simulink model "MPSK_basemodem"  (Simulink 9.2)
settings: Solver=VariableStepDiscrete  StartTime=0.0  StopTime=10  FixedStep=1/100000  RelTol=1e-3  AbsTol=1e-6
PreLoadFcn:
  | M=16;
libraries: commutil2 x2, commsink2 x2, commdigbbndpm3 x2, commchan3 x1, commrandsrc2 x1
settings Model: Creator=amoura  LastModifiedBy=nox
settings SolverCC: AutoScaleAbsTol=off
settings DataIOCC: LimitDataPoints=off
settings OptimizationCC: BlockReduction=off  BooleanDataType=off  ExpressionDepthLimit=2147483647  InitFltsAndDblsToZero=on
settings DebuggingCC: SaveWithParameterizedLinksMsg=none  SignalResolutionControl=TryResolveAllWithWarning  MultiTaskDSMMsg=warning  MultiTaskCondExecSysMsg=none
settings HardwareCC: TargetUnknown=on
settings RTWCC: TemplateMakefile=grt_unix.tmf
settings GRTTargetCC: TargetFcnLib=ansi_tfl_tmw.mat  ModelReferenceCompliant=off  MatFileLogging=off

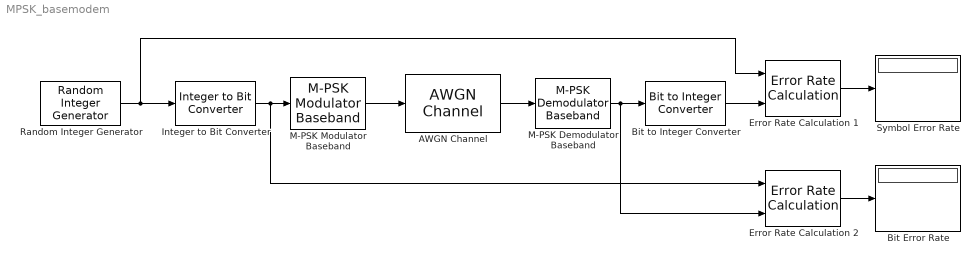
== system MPSK_basemodem ==
  AWGN Channel : commchan3/AWGN Channel  InputProcessing=Columns as channels (frame based)  seed=67  noiseMode="Signal to noise ratio  (Es/No)"  EbNodB=9.21  EsNodB=8  SNRdB=10  bitsPerSym=3  Ps=1  Tsym=1/1000  variance=1
  Bit Error Rate : Display
  Bit to Integer Converter : commutil2/Bit to Integer Converter  nbits=log2(M)  bitOrder=MSB first  signedOutputValues=Unsigned  outDtype=Inherit via internal rule  outDtypeSigned=Inherit via internal rule
  Error Rate Calculation 1 : commsink2/Error Rate Calculation  N=0  st_delay=0  cp_mode=Entire frame  subframe=[]  PMode=Port  WsName=ErrorVec  RsMode2=off  stop=off  numErr=100  maxBits=1e6
  Error Rate Calculation 2 : commsink2/Error Rate Calculation  N=0  st_delay=0  cp_mode=Entire frame  subframe=[]  PMode=Port  WsName=ErrorVec  RsMode2=off  stop=off  numErr=100  maxBits=1e6
  Integer to Bit Converter : commutil2/Integer to Bit Converter  nbits=log2(M)  signedInputValues=Unsigned  bitOrder=MSB first  outDtype=Inherit via internal rule
  M-PSK Demodulator Baseband : commdigbbndpm3/M-PSK Demodulator Baseband  M=M  OutType=Bit  DecType=Hard decision  VarSource=Dialog  Variance=1  Dec=Gray  Mapping=[0:7]  Ph=0  outDtype1=Inherit via internal rule  outDtype2=double  derotateFactorWordLen=16  derotateFactorDataTypeStr=Inherit: Same word length as input  derotateFactorLastDataTypeStr=Inherit: Same word length as input
      settings: SourceProductName=Communications System Toolbox
  M-PSK Modulator Baseband : commdigbbndpm3/M-PSK Modulator Baseband  M=M  InType=Bit  Enc=Gray  Mapping=[0:7]  Ph=0  outDtype=double  outWordLen=16  outUDDataType=sfix(16)  outFracLenMode=Best precision  outFracLen=15  outDataTypeStr=double  outLastDataTypeStr=double
      settings: SourceProductName=Communications System Toolbox
  Random Integer Generator : commrandsrc2/Random Integer Generator  mul=M  seed=529558  Ts=1/1000  frameBased=on  sampPerFrame=100  orient=off  outDataType=double
  "Symbol Error Rate " : Display
  wires:
  Error Rate Calculation 1/1 -> "Symbol Error Rate "/1
  Random Integer Generator/1 -> Error Rate Calculation 1/1, Integer to Bit Converter/1
  AWGN Channel/1 -> M-PSK Demodulator Baseband/1
  M-PSK Modulator Baseband/1 -> AWGN Channel/1
  Integer to Bit Converter/1 -> M-PSK Modulator Baseband/1, Error Rate Calculation 2/1
  M-PSK Demodulator Baseband/1 -> Bit to Integer Converter/1, Error Rate Calculation 2/2
  Bit to Integer Converter/1 -> Error Rate Calculation 1/2
  Error Rate Calculation 2/1 -> Bit Error Rate/1
